simulink model "pfb_fir_16k_4tap_v3_core"  (Simulink 7.8)
settings: Solver=ode45  StartTime=0.0  StopTime=10.0  RelTol=1e-3
libraries: xbsIndex_r4 x287, casper_library_misc x8
(part 1 of 9)
settings Model: Creator=dan  LastModifiedBy=dan
settings DebuggingCC: FcnCallInpInsideContextMsg=Use local settings  StrictBusMsg=Warning

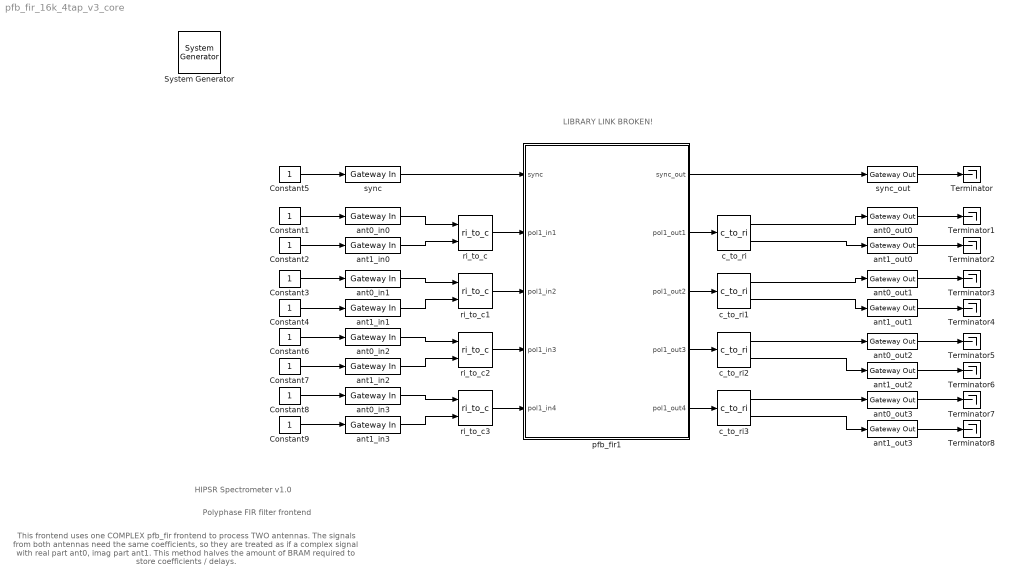
== system pfb_fir_16k_4tap_v3_core ==
  note: Polyphase FIR filter frontend
  note: HIPSR Spectrometer v1.0
  note: This frontend uses one COMPLEX pfb_fir frontend to process TWO antennas.
      | The signals from both antennas need the same coefficients, so they are
      | treated as if a complex signal with real part ant0, imag part ant1.
      | This method halves the amount of BRAM required to store coefficients / delays.
  note: LIBRARY LINK BROKEN!
  " System Generator" : xbsIndex_r4/ System Generator  Tag=genX  xilinxfamily=virtex5  part=xc5vsx95t  speed=-1  package=ff1136  synthesis_tool=XST  clock_wrapper=Clock Enables  directory=/designs/dan/parkes/bb/xb_pfb_fir_16k_4tap_core  proj_type=Project Navigator  Synth_file=XST Defaults  Impl_file=ISE Defaults  testbench=off  simulink_period=1  sysclk_period=10  dcm_input_clock_period=10  incr_netlist=off  trim_vbits=Everywhere in SubSystem  dbl_ovrd=According to Block Masks  core_generation=According to Block Masks  run_coregen=off  deprecated_control=off  eval_field=0  block_type=sysgen
      settings: block_version=11.4
  Constant{1..9} (9 alike) : Constant
  Terminator{,1..8} (9 alike) : Terminator
  ant0_in{0..3} (4 alike) : xbsIndex_r4/Gateway In  gui_display_data_type=Fixed-point  arith_type="Signed  (2's comp)"  n_bits=8  bin_pt=7  preci_type=Single  exp_width=8  frac_width=24  quantization="Round  (unbiased: +/- Inf)"  overflow=Saturate  period=1  dbl_ovrd=off  timing_constraint=None  locs_specified=off  LOCs={}  inherit_from_input=off  UseAsADC=off  ADCChannel='1'  hdl_port=on  block_type=gatewayin
      settings: infoedit="Gateway in block.  Converts inputs of type Simulink integer, double and fixed point to  Xilinx fixed point type.<br><br>Hardware notes:  In hardware these blocks become top level input ports."  block_version=11.4
  ant0_out{0..3} (4 alike) : xbsIndex_r4/Gateway Out  inherit_from_input=off  hdl_port=on  timing_constraint=None  locs_specified=off  LOCs={}  UseAsDAC=off  DACChannel='1'  block_type=gatewayout
      settings: infoedit="Gateway out block.  Converts Xilinx fixed point inputs into ouputs of type Simulink integer, double, or fixed point.<br><br>Hardware notes:  In hardware these blocks become top level output ports or are discarded, depending on how they are configured."  block_version=11.4
  ant1_in{0..3} (4 alike) : xbsIndex_r4/Gateway In  gui_display_data_type=Fixed-point  arith_type="Signed  (2's comp)"  n_bits=8  bin_pt=7  preci_type=Single  exp_width=8  frac_width=24  quantization="Round  (unbiased: +/- Inf)"  overflow=Saturate  period=1  dbl_ovrd=off  timing_constraint=None  locs_specified=off  LOCs={}  inherit_from_input=off  UseAsADC=off  ADCChannel='1'  hdl_port=on  block_type=gatewayin
      settings: infoedit="Gateway in block.  Converts inputs of type Simulink integer, double and fixed point to  Xilinx fixed point type.<br><br>Hardware notes:  In hardware these blocks become top level input ports."  block_version=11.4
  ant1_out{0..3} (4 alike) : xbsIndex_r4/Gateway Out  inherit_from_input=off  hdl_port=on  timing_constraint=None  locs_specified=off  LOCs={}  UseAsDAC=off  DACChannel='1'  block_type=gatewayout
      settings: infoedit="Gateway out block.  Converts Xilinx fixed point inputs into ouputs of type Simulink integer, double, or fixed point.<br><br>Hardware notes:  In hardware these blocks become top level output ports or are discarded, depending on how they are configured."  block_version=11.4
  c_to_ri{,1..3} (4 alike) : casper_library_misc/c_to_ri  n_bits=18  bin_pt=17
  pfb_fir1 : Subsystem  AncestorBlock=xblocks_library_pfbs/pfb_fir  mask(pfb_fir){PFBSize=14, TotalTaps=4, WindowType=hamming, n_inputs=2, MakeBiplex=off, BitWidthIn=8, BitWidthOut=18, CoeffBitWidth=18, CoeffDistMem=off, add_latency=2, mult_latency=3, bram_latency=3, quantization=Round  (unbiased: +/- Inf), fwidth=1, specify_mult=off, mult_spec=[2                                      2]}
      mask prompts: PFBSize "Size of PFB: (2^? pnts)"; TotalTaps "Total Number of Taps:"; WindowType "Windowing Function:"; n_inputs "Number of Simultaneous Inputs: (2^?)"; MakeBiplex "Make Biplex"; BitWidthIn "Input Bitwidth:"; BitWidthOut "Output Bitwidth:"; CoeffBitWidth "Coefficient Bitwidth:"; CoeffDistMem "Use Distributed Memory for Coeffs"; add_latency "Add Latency"; mult_latency "Mult Latency"; bram_latency "BRAM Latency"; quantization "Quantization Behavior"; fwidth "Bin Width Scaling (normal=1)"; specify_mult "Specify multiplier use (behavioral if not specified)"; mult_spec "Multiplier specification (0=core, 1=embedded, 2=behavioural) (left=1st tap)"
      mask init:
      | config.source = str2func('pfb_fir_init_xblock');
      | config.toplevel = gcb;
      | config.depend = get_dependlist('pfb_fir');
      | set_param(gcb,'LinkStatus','inactive');
      | xBlock(config,{config.toplevel, ...
      |     'PFBSize', PFBSize, ...
      |     'TotalTaps', TotalTaps, ...
      |     'WindowType', WindowType, ...
      |     'n_inputs', n_inputs, ...
      |     'MakeBiplex', MakeBiplex, ...
      |     'BitWidthIn', BitWidthIn, ...
      |     'BitWidthOut', BitWidthOut, ...
      |     'CoeffBitWidth', CoeffBitWidth, ...
      |     'CoeffDistMem', CoeffDistMem, ...
      |     'add_latency', add_latency, ...
      |     'mult_latency', mult_latency, ...
      |     'bram_latency', bram_latency, ...
      |     'quantization', quantization, ...
      |     'fwidth', fwidth,...
      |     'specify_mult', specify_mult,...
      |     'mult_spec', mult_spec});
      settings: AttributesFormatString=taps=4, add_latency=2
      mask Help: eval('xlWeb(''http://casper.berkeley.edu/wiki/Pfb_fir'')')
      mask StyleString: edit,edit,popup(bartlett|barthannwin|blackman|blackmanharris|bohamwin|chebwin|flattopwin|gausswin|hamming|hann|kaiser|nuttallwin|parzenwin|rectwin|tukeywin|triang|userwindow),edit,checkbox,edit,edit,edit,checkbox,edit,edit,edit,popup(Truncate|Round  (unbiased: +/- Inf)|Round  (unbiased: Even Values)),edit,checkbox,edit
      mask CallbackString:
      | |%num_taps = eval(get_param(gcb, 'TotalTaps'));
      | %old_vec = eval(get_param(gcb, 'mult_spec'));
      | 
      | %vec = 2.*ones(1,num_taps);
      | %old_size = length(old_vec);
      | 
      | %if(old_size <= num_taps),
      | %   new_size = old_size;
      | %else,
      | %    new_size = num_taps;
      | %end
      | 
      | %for n = 1:new_size, vec(n) = old_vec(n); end
      | %set_param(gcb, 'mult_spec', mat2str(vec));||||||||||||%num_taps = eval(get_param(gcb, 'TotalTaps'));
      | %old_vec = eval(get_param(gcb, 'mult_spec'));
      | 
      | %vec = 2.*ones(1,num_taps);
      | %old_size = length(old_vec);
      | 
      | %if(old_size <= num_taps),
      | %    new_size = old_size;
      | %else,
      | %    new_size = num_taps;
      | %end
      | 
      | %for n = 1:new_size, vec(n) = old_vec(n); end
      | %set_param(gcb, 'mult_spec', mat2str(vec));|%specify_mult = get_param(gcb,'specify_mult');
      | %if( strcmp(specify_mult,'off')),
      | %    set_param(gcb, 'MaskEnables', {'on','on','on','on','on','on','on','on','on','on','on','on','on','on','on','off'});
      | %else
      | %    set_param(gcb, 'MaskEnables', {'on','on','on','on','on','on','on','on','on','on','on','on','on','on','on','on'});
      | %end
      | 
      | |%specify_mult = get_param(gcb,'specify_mult');
      | %if( strcmp(specify_mult,'off')),
      | %    set_param(gcb, 'MaskEnables', {'on','on','on','on','on','on','on','on','on','on','on','on','on','on','on','off'});
      | %else
      | %    set_param(gcb, 'MaskEnables', {'on','on','on','on','on','on','on','on','on','on','on','on','on','on','on','on'});
      | %end
  ri_to_c{,1..3} (4 alike) : casper_library_misc/ri_to_c
  sync : xbsIndex_r4/Gateway In  gui_display_data_type=Fixed-point  arith_type=Boolean  n_bits=16  bin_pt=14  preci_type=Single  exp_width=8  frac_width=24  quantization="Round  (unbiased: +/- Inf)"  overflow=Saturate  period=1  dbl_ovrd=off  timing_constraint=None  locs_specified=off  LOCs={}  inherit_from_input=off  UseAsADC=off  ADCChannel='1'  hdl_port=on  block_type=gatewayin
      settings: infoedit="Gateway in block.  Converts inputs of type Simulink integer, double and fixed point to  Xilinx fixed point type.<br><br>Hardware notes:  In hardware these blocks become top level input ports."  block_version=11.4
  sync_out : xbsIndex_r4/Gateway Out  inherit_from_input=off  hdl_port=on  timing_constraint=None  locs_specified=off  LOCs={}  UseAsDAC=off  DACChannel='1'  block_type=gatewayout
      settings: infoedit="Gateway out block.  Converts Xilinx fixed point inputs into ouputs of type Simulink integer, double, or fixed point.<br><br>Hardware notes:  In hardware these blocks become top level output ports or are discarded, depending on how they are configured."  block_version=11.4
  wires:
  sync/1 -> pfb_fir1/1(sync)
  ri_to_c/1 -> pfb_fir1/2(pol1_in1)
  ri_to_c1/1 -> pfb_fir1/3(pol1_in2)
  ant0_in0/1 -> ri_to_c/1
  Constant5/1 -> sync/1
  Constant1/1 -> ant0_in0/1
  ant1_in0/1 -> ri_to_c/2
  ant0_in1/1 -> ri_to_c1/1
  ant1_in1/1 -> ri_to_c1/2
  Constant4/1 -> ant1_in1/1
  Constant3/1 -> ant0_in1/1
  Constant2/1 -> ant1_in0/1
  pfb_fir1/2(pol1_out1) -> c_to_ri/1
  pfb_fir1/3(pol1_out2) -> c_to_ri1/1
  sync_out/1 -> Terminator/1
  ant1_out0/1 -> Terminator2/1
  ant0_out0/1 -> Terminator1/1
  ant0_in2/1 -> ri_to_c2/1
  ant1_in2/1 -> ri_to_c2/2
  Constant7/1 -> ant1_in2/1
  Constant6/1 -> ant0_in2/1
  ant0_in3/1 -> ri_to_c3/1
  ant1_in3/1 -> ri_to_c3/2
  Constant9/1 -> ant1_in3/1
  Constant8/1 -> ant0_in3/1
  ri_to_c2/1 -> pfb_fir1/4(pol1_in3)
  ri_to_c3/1 -> pfb_fir1/5(pol1_in4)
  pfb_fir1/1(sync_out) -> sync_out/1
  ant1_out1/1 -> Terminator4/1
  ant0_out1/1 -> Terminator3/1
  ant1_out2/1 -> Terminator6/1
  ant0_out2/1 -> Terminator5/1
  ant1_out3/1 -> Terminator8/1
  ant0_out3/1 -> Terminator7/1
  c_to_ri/1 -> ant0_out0/1
  c_to_ri/2 -> ant1_out0/1
  c_to_ri1/1 -> ant0_out1/1
  c_to_ri1/2 -> ant1_out1/1
  c_to_ri2/1 -> ant0_out2/1
  c_to_ri2/2 -> ant1_out2/1
  c_to_ri3/1 -> ant0_out3/1
  c_to_ri3/2 -> ant1_out3/1
  pfb_fir1/4(pol1_out3) -> c_to_ri2/1
  pfb_fir1/5(pol1_out4) -> c_to_ri3/1

== system pfb_fir_16k_4tap_v3_core/pfb_fir1 ==
  sync : Inport
  pol1_in1 : Inport  Port=2
  pol1_in2 : Inport  Port=3
  pol1_in3 : Inport  Port=4
  pol1_in4 : Inport  Port=5
  pfb_row_11 : Subsystem
  pfb_row_12 : Subsystem
  pfb_row_13 : Subsystem
  pfb_row_14 : Subsystem
  sync_out : Outport
  pol1_out1 : Outport  Port=2
  pol1_out2 : Outport  Port=3
  pol1_out3 : Outport  Port=4
  pol1_out4 : Outport  Port=5
  wires:
  sync/1 -> pfb_row_14/2(sync), pfb_row_13/2(sync), pfb_row_12/2(sync), pfb_row_11/2(sync)
  pfb_row_14/2(out) -> pol1_out4/1
  pol1_in4/1 -> pfb_row_14/1(din)
  pfb_row_13/2(out) -> pol1_out3/1
  pol1_in3/1 -> pfb_row_13/1(din)
  pfb_row_12/2(out) -> pol1_out2/1
  pol1_in2/1 -> pfb_row_12/1(din)
  pfb_row_11/2(out) -> pol1_out1/1
  pfb_row_11/1(sync_out) -> sync_out/1
  pol1_in1/1 -> pfb_row_11/1(din)

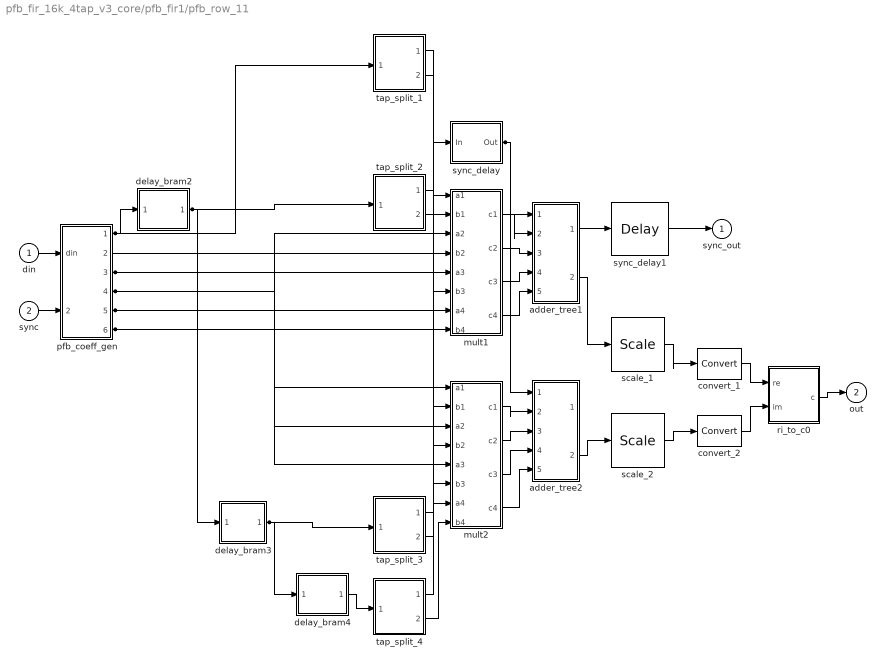
== system pfb_fir_16k_4tap_v3_core/pfb_fir1/pfb_row_11 ==
  din : Inport
  sync : Inport  Port=2
  adder_tree1 : Subsystem
  adder_tree2 : Subsystem
  convert_1 : xbsIndex_r4/Convert  gui_display_data_type=Fixed-point  arith_type="Signed  (2's comp)"  n_bits=18  bin_pt=17  float_type=Single  exp_bits=8  fraction_bits=24  quantization="Round  (unbiased: +/- Inf)"  overflow=Saturate  en=off  latency=3  dbl_ovrd=off  pipeline=on  block_type=convert
  convert_2 : xbsIndex_r4/Convert  gui_display_data_type=Fixed-point  arith_type="Signed  (2's comp)"  n_bits=18  bin_pt=17  float_type=Single  exp_bits=8  fraction_bits=24  quantization="Round  (unbiased: +/- Inf)"  overflow=Saturate  en=off  latency=3  dbl_ovrd=off  pipeline=on  block_type=convert
  delay_bram2 : Subsystem
  delay_bram3 : Subsystem
  delay_bram4 : Subsystem
  mult1 : Subsystem
  mult2 : Subsystem
  pfb_coeff_gen : Subsystem
      settings: AttributesFormatString=PFBSize=14, n_inputs=2, taps=4
  ri_to_c0 : Subsystem
  scale_1 : xbsIndex_r4/Scale  scale_factor=-3  dbl_ovrd=off  block_type=scale
  scale_2 : xbsIndex_r4/Scale  scale_factor=-3  dbl_ovrd=off  block_type=scale
  sync_delay : Subsystem
  sync_delay1 : xbsIndex_r4/Delay  rst=off  infoeditControl=Selection of Reset will increase slice count due to use of real FFs and instead of SRLs  en=off  latency=3  dbl_ovrd=off  reg_retiming=off  block_type=delay
  tap_split_1 : Subsystem
      settings: AttributesFormatString=Fix_8_7
  tap_split_2 : Subsystem
      settings: AttributesFormatString=Fix_8_7
  tap_split_3 : Subsystem
      settings: AttributesFormatString=Fix_8_7
  tap_split_4 : Subsystem
      settings: AttributesFormatString=Fix_8_7
  sync_out : Outport
  out : Outport  Port=2
  wires:
  pfb_coeff_gen/1(dout) -> tap_split_1/1(inport), delay_bram2/1(din_1_1)
  delay_bram2/1(dout_1_1) -> tap_split_2/1(inport), delay_bram3/1(din_1_1)
  delay_bram3/1(dout_1_1) -> tap_split_3/1(inport), delay_bram4/1(din_1_1)
  pfb_coeff_gen/3(coeffs1) -> mult2/1(a1), mult1/1(a1)
  pfb_coeff_gen/4(coeffs2) -> mult2/3(a2), mult1/3(a2)
  pfb_coeff_gen/5(coeffs3) -> mult2/5(a3), mult1/5(a3)
  pfb_coeff_gen/6(coeffs4) -> mult2/7(a4), mult1/7(a4)
  sync_delay/1(Out) -> adder_tree2/1(sync), adder_tree1/1(sync)
  ri_to_c0/1(c) -> out/1
  convert_2/1 -> ri_to_c0/2(im)
  convert_1/1 -> ri_to_c0/1(re)
  scale_2/1 -> convert_2/1
  adder_tree2/2(dout) -> scale_2/1
  mult2/4(c4) -> adder_tree2/5(din_4)
  mult2/3(c3) -> adder_tree2/4(din_3)
  mult2/2(c2) -> adder_tree2/3(din_2)
  mult2/1(c1) -> adder_tree2/2(din_1)
  tap_split_4/2(outport2) -> mult2/8(b4)
  tap_split_3/2(outport2) -> mult2/6(b3)
  tap_split_2/2(outport2) -> mult2/4(b2)
  tap_split_1/2(outport2) -> mult2/2(b1)
  sync_delay1/1 -> sync_out/1
  adder_tree1/1(sync_out) -> sync_delay1/1
  scale_1/1 -> convert_1/1
  adder_tree1/2(dout) -> scale_1/1
  mult1/4(c4) -> adder_tree1/5(din_4)
  mult1/3(c3) -> adder_tree1/4(din_3)
  mult1/2(c2) -> adder_tree1/3(din_2)
  mult1/1(c1) -> adder_tree1/2(din_1)
  tap_split_4/1(outport1) -> mult1/8(b4)
  tap_split_3/1(outport1) -> mult1/6(b3)
  tap_split_2/1(outport1) -> mult1/4(b2)
  tap_split_1/1(outport1) -> mult1/2(b1)
  delay_bram4/1(dout_1_1) -> tap_split_4/1(inport)
  pfb_coeff_gen/2(sync_out) -> sync_delay/1(In)
  sync/1 -> pfb_coeff_gen/2(sync)
  din/1 -> pfb_coeff_gen/1(din)

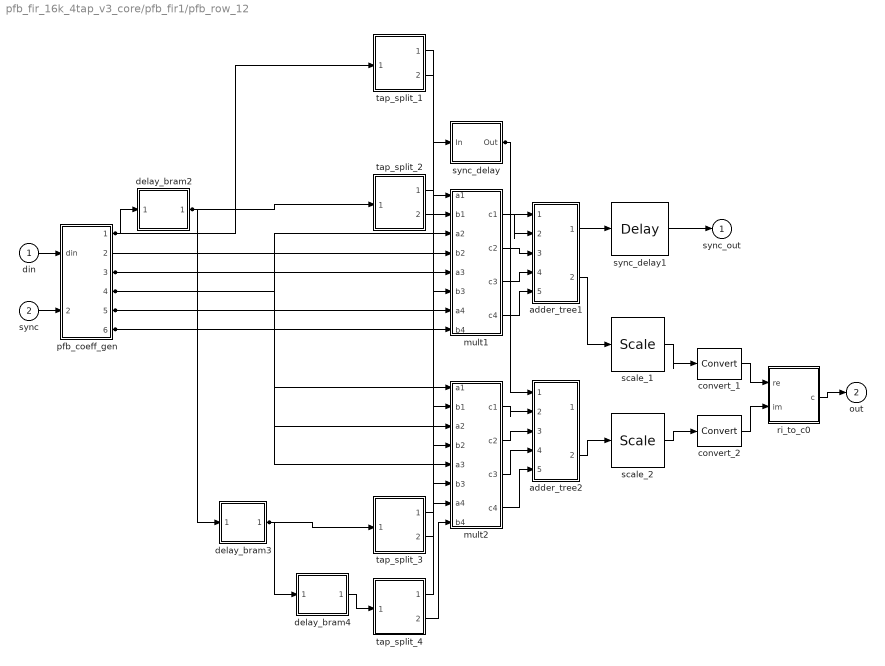
== system pfb_fir_16k_4tap_v3_core/pfb_fir1/pfb_row_12 ==
  din : Inport
  sync : Inport  Port=2
  adder_tree1 : Subsystem
  adder_tree2 : Subsystem
  convert_1 : xbsIndex_r4/Convert  gui_display_data_type=Fixed-point  arith_type="Signed  (2's comp)"  n_bits=18  bin_pt=17  float_type=Single  exp_bits=8  fraction_bits=24  quantization="Round  (unbiased: +/- Inf)"  overflow=Saturate  en=off  latency=3  dbl_ovrd=off  pipeline=on  block_type=convert
  convert_2 : xbsIndex_r4/Convert  gui_display_data_type=Fixed-point  arith_type="Signed  (2's comp)"  n_bits=18  bin_pt=17  float_type=Single  exp_bits=8  fraction_bits=24  quantization="Round  (unbiased: +/- Inf)"  overflow=Saturate  en=off  latency=3  dbl_ovrd=off  pipeline=on  block_type=convert
  delay_bram2 : Subsystem
  delay_bram3 : Subsystem
  delay_bram4 : Subsystem
  mult1 : Subsystem
  mult2 : Subsystem
  pfb_coeff_gen : Subsystem
      settings: AttributesFormatString=PFBSize=14, n_inputs=2, taps=4
  ri_to_c0 : Subsystem
  scale_1 : xbsIndex_r4/Scale  scale_factor=-3  dbl_ovrd=off  block_type=scale
  scale_2 : xbsIndex_r4/Scale  scale_factor=-3  dbl_ovrd=off  block_type=scale
  sync_delay : Subsystem
  sync_delay1 : xbsIndex_r4/Delay  rst=off  infoeditControl=Selection of Reset will increase slice count due to use of real FFs and instead of SRLs  en=off  latency=3  dbl_ovrd=off  reg_retiming=off  block_type=delay
  tap_split_1 : Subsystem
      settings: AttributesFormatString=Fix_8_7
  tap_split_2 : Subsystem
      settings: AttributesFormatString=Fix_8_7
  tap_split_3 : Subsystem
      settings: AttributesFormatString=Fix_8_7
  tap_split_4 : Subsystem
      settings: AttributesFormatString=Fix_8_7
  sync_out : Outport
  out : Outport  Port=2
  wires:
  pfb_coeff_gen/1(dout) -> tap_split_1/1(inport), delay_bram2/1(din_1_1)
  delay_bram2/1(dout_1_1) -> tap_split_2/1(inport), delay_bram3/1(din_1_1)
  delay_bram3/1(dout_1_1) -> tap_split_3/1(inport), delay_bram4/1(din_1_1)
  pfb_coeff_gen/3(coeffs1) -> mult2/1(a1), mult1/1(a1)
  pfb_coeff_gen/4(coeffs2) -> mult2/3(a2), mult1/3(a2)
  pfb_coeff_gen/5(coeffs3) -> mult2/5(a3), mult1/5(a3)
  pfb_coeff_gen/6(coeffs4) -> mult2/7(a4), mult1/7(a4)
  sync_delay/1(Out) -> adder_tree2/1(sync), adder_tree1/1(sync)
  ri_to_c0/1(c) -> out/1
  convert_2/1 -> ri_to_c0/2(im)
  convert_1/1 -> ri_to_c0/1(re)
  scale_2/1 -> convert_2/1
  adder_tree2/2(dout) -> scale_2/1
  mult2/4(c4) -> adder_tree2/5(din_4)
  mult2/3(c3) -> adder_tree2/4(din_3)
  mult2/2(c2) -> adder_tree2/3(din_2)
  mult2/1(c1) -> adder_tree2/2(din_1)
  tap_split_4/2(outport2) -> mult2/8(b4)
  tap_split_3/2(outport2) -> mult2/6(b3)
  tap_split_2/2(outport2) -> mult2/4(b2)
  tap_split_1/2(outport2) -> mult2/2(b1)
  sync_delay1/1 -> sync_out/1
  adder_tree1/1(sync_out) -> sync_delay1/1
  scale_1/1 -> convert_1/1
  adder_tree1/2(dout) -> scale_1/1
  mult1/4(c4) -> adder_tree1/5(din_4)
  mult1/3(c3) -> adder_tree1/4(din_3)
  mult1/2(c2) -> adder_tree1/3(din_2)
  mult1/1(c1) -> adder_tree1/2(din_1)
  tap_split_4/1(outport1) -> mult1/8(b4)
  tap_split_3/1(outport1) -> mult1/6(b3)
  tap_split_2/1(outport1) -> mult1/4(b2)
  tap_split_1/1(outport1) -> mult1/2(b1)
  delay_bram4/1(dout_1_1) -> tap_split_4/1(inport)
  pfb_coeff_gen/2(sync_out) -> sync_delay/1(In)
  sync/1 -> pfb_coeff_gen/2(sync)
  din/1 -> pfb_coeff_gen/1(din)

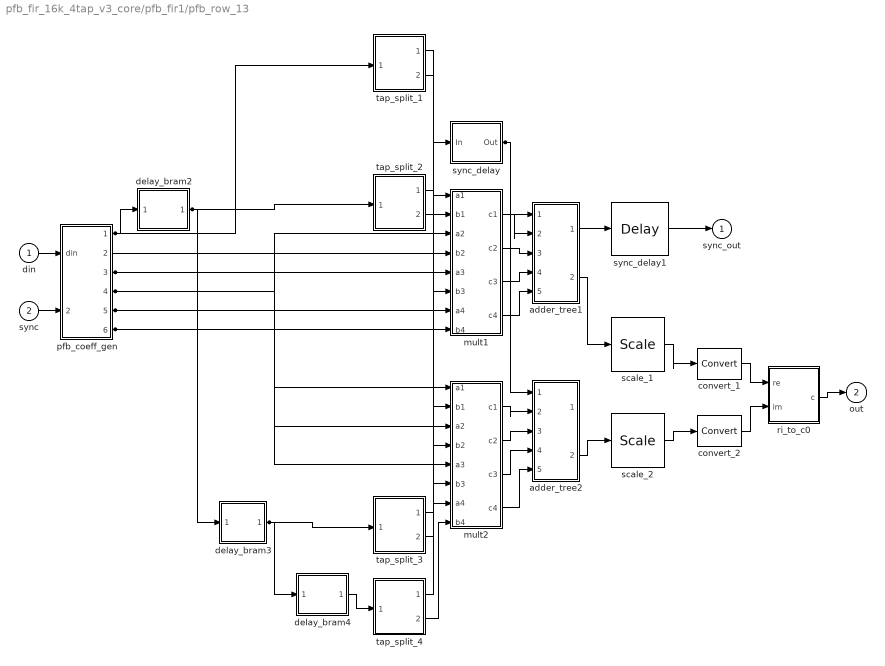
== system pfb_fir_16k_4tap_v3_core/pfb_fir1/pfb_row_13 ==
  din : Inport
  sync : Inport  Port=2
  adder_tree1 : Subsystem
  adder_tree2 : Subsystem
  convert_1 : xbsIndex_r4/Convert  gui_display_data_type=Fixed-point  arith_type="Signed  (2's comp)"  n_bits=18  bin_pt=17  float_type=Single  exp_bits=8  fraction_bits=24  quantization="Round  (unbiased: +/- Inf)"  overflow=Saturate  en=off  latency=3  dbl_ovrd=off  pipeline=on  block_type=convert
  convert_2 : xbsIndex_r4/Convert  gui_display_data_type=Fixed-point  arith_type="Signed  (2's comp)"  n_bits=18  bin_pt=17  float_type=Single  exp_bits=8  fraction_bits=24  quantization="Round  (unbiased: +/- Inf)"  overflow=Saturate  en=off  latency=3  dbl_ovrd=off  pipeline=on  block_type=convert
  delay_bram2 : Subsystem
  delay_bram3 : Subsystem
  delay_bram4 : Subsystem
  mult1 : Subsystem
  mult2 : Subsystem
  pfb_coeff_gen : Subsystem
      settings: AttributesFormatString=PFBSize=14, n_inputs=2, taps=4
  ri_to_c0 : Subsystem
  scale_1 : xbsIndex_r4/Scale  scale_factor=-3  dbl_ovrd=off  block_type=scale
  scale_2 : xbsIndex_r4/Scale  scale_factor=-3  dbl_ovrd=off  block_type=scale
  sync_delay : Subsystem
  sync_delay1 : xbsIndex_r4/Delay  rst=off  infoeditControl=Selection of Reset will increase slice count due to use of real FFs and instead of SRLs  en=off  latency=3  dbl_ovrd=off  reg_retiming=off  block_type=delay
  tap_split_1 : Subsystem
      settings: AttributesFormatString=Fix_8_7
  tap_split_2 : Subsystem
      settings: AttributesFormatString=Fix_8_7
  tap_split_3 : Subsystem
      settings: AttributesFormatString=Fix_8_7
  tap_split_4 : Subsystem
      settings: AttributesFormatString=Fix_8_7
  sync_out : Outport
  out : Outport  Port=2
  wires:
  pfb_coeff_gen/1(dout) -> tap_split_1/1(inport), delay_bram2/1(din_1_1)
  delay_bram2/1(dout_1_1) -> tap_split_2/1(inport), delay_bram3/1(din_1_1)
  delay_bram3/1(dout_1_1) -> tap_split_3/1(inport), delay_bram4/1(din_1_1)
  pfb_coeff_gen/3(coeffs1) -> mult2/1(a1), mult1/1(a1)
  pfb_coeff_gen/4(coeffs2) -> mult2/3(a2), mult1/3(a2)
  pfb_coeff_gen/5(coeffs3) -> mult2/5(a3), mult1/5(a3)
  pfb_coeff_gen/6(coeffs4) -> mult2/7(a4), mult1/7(a4)
  sync_delay/1(Out) -> adder_tree2/1(sync), adder_tree1/1(sync)
  ri_to_c0/1(c) -> out/1
  convert_2/1 -> ri_to_c0/2(im)
  convert_1/1 -> ri_to_c0/1(re)
  scale_2/1 -> convert_2/1
  adder_tree2/2(dout) -> scale_2/1
  mult2/4(c4) -> adder_tree2/5(din_4)
  mult2/3(c3) -> adder_tree2/4(din_3)
  mult2/2(c2) -> adder_tree2/3(din_2)
  mult2/1(c1) -> adder_tree2/2(din_1)
  tap_split_4/2(outport2) -> mult2/8(b4)
  tap_split_3/2(outport2) -> mult2/6(b3)
  tap_split_2/2(outport2) -> mult2/4(b2)
  tap_split_1/2(outport2) -> mult2/2(b1)
  sync_delay1/1 -> sync_out/1
  adder_tree1/1(sync_out) -> sync_delay1/1
  scale_1/1 -> convert_1/1
  adder_tree1/2(dout) -> scale_1/1
  mult1/4(c4) -> adder_tree1/5(din_4)
  mult1/3(c3) -> adder_tree1/4(din_3)
  mult1/2(c2) -> adder_tree1/3(din_2)
  mult1/1(c1) -> adder_tree1/2(din_1)
  tap_split_4/1(outport1) -> mult1/8(b4)
  tap_split_3/1(outport1) -> mult1/6(b3)
  tap_split_2/1(outport1) -> mult1/4(b2)
  tap_split_1/1(outport1) -> mult1/2(b1)
  delay_bram4/1(dout_1_1) -> tap_split_4/1(inport)
  pfb_coeff_gen/2(sync_out) -> sync_delay/1(In)
  sync/1 -> pfb_coeff_gen/2(sync)
  din/1 -> pfb_coeff_gen/1(din)

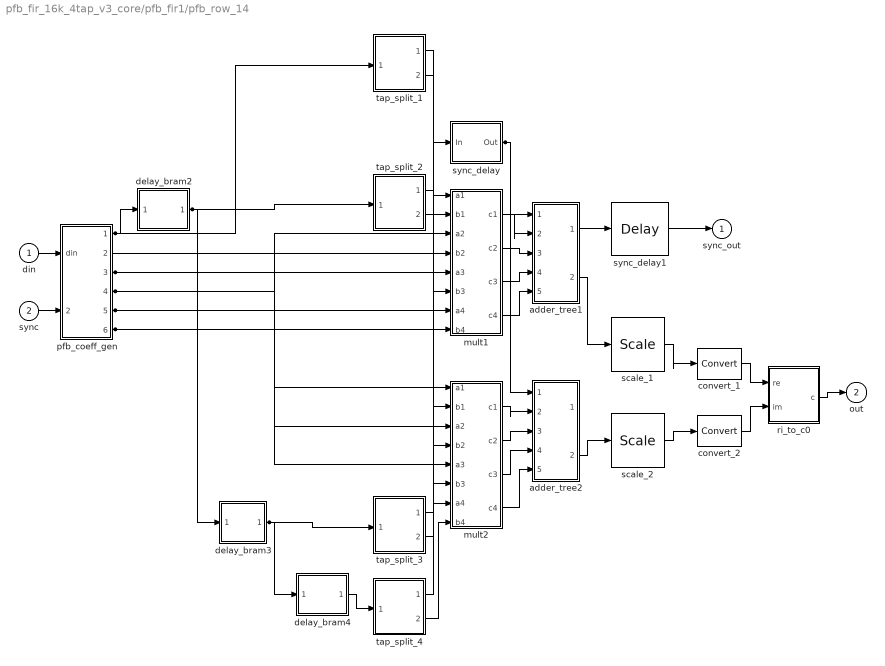
== system pfb_fir_16k_4tap_v3_core/pfb_fir1/pfb_row_14 ==
  din : Inport
  sync : Inport  Port=2
  adder_tree1 : Subsystem
  adder_tree2 : Subsystem
  convert_1 : xbsIndex_r4/Convert  gui_display_data_type=Fixed-point  arith_type="Signed  (2's comp)"  n_bits=18  bin_pt=17  float_type=Single  exp_bits=8  fraction_bits=24  quantization="Round  (unbiased: +/- Inf)"  overflow=Saturate  en=off  latency=3  dbl_ovrd=off  pipeline=on  block_type=convert
  convert_2 : xbsIndex_r4/Convert  gui_display_data_type=Fixed-point  arith_type="Signed  (2's comp)"  n_bits=18  bin_pt=17  float_type=Single  exp_bits=8  fraction_bits=24  quantization="Round  (unbiased: +/- Inf)"  overflow=Saturate  en=off  latency=3  dbl_ovrd=off  pipeline=on  block_type=convert
  delay_bram2 : Subsystem
  delay_bram3 : Subsystem
  delay_bram4 : Subsystem
  mult1 : Subsystem
  mult2 : Subsystem
  pfb_coeff_gen : Subsystem
      settings: AttributesFormatString=PFBSize=14, n_inputs=2, taps=4
  ri_to_c0 : Subsystem
  scale_1 : xbsIndex_r4/Scale  scale_factor=-3  dbl_ovrd=off  block_type=scale
  scale_2 : xbsIndex_r4/Scale  scale_factor=-3  dbl_ovrd=off  block_type=scale
  sync_delay : Subsystem
  sync_delay1 : xbsIndex_r4/Delay  rst=off  infoeditControl=Selection of Reset will increase slice count due to use of real FFs and instead of SRLs  en=off  latency=3  dbl_ovrd=off  reg_retiming=off  block_type=delay
  tap_split_1 : Subsystem
      settings: AttributesFormatString=Fix_8_7
  tap_split_2 : Subsystem
      settings: AttributesFormatString=Fix_8_7
  tap_split_3 : Subsystem
      settings: AttributesFormatString=Fix_8_7
  tap_split_4 : Subsystem
      settings: AttributesFormatString=Fix_8_7
  sync_out : Outport
  out : Outport  Port=2
  wires:
  pfb_coeff_gen/1(dout) -> tap_split_1/1(inport), delay_bram2/1(din_1_1)
  delay_bram2/1(dout_1_1) -> tap_split_2/1(inport), delay_bram3/1(din_1_1)
  delay_bram3/1(dout_1_1) -> tap_split_3/1(inport), delay_bram4/1(din_1_1)
  pfb_coeff_gen/3(coeffs1) -> mult2/1(a1), mult1/1(a1)
  pfb_coeff_gen/4(coeffs2) -> mult2/3(a2), mult1/3(a2)
  pfb_coeff_gen/5(coeffs3) -> mult2/5(a3), mult1/5(a3)
  pfb_coeff_gen/6(coeffs4) -> mult2/7(a4), mult1/7(a4)
  sync_delay/1(Out) -> adder_tree2/1(sync), adder_tree1/1(sync)
  ri_to_c0/1(c) -> out/1
  convert_2/1 -> ri_to_c0/2(im)
  convert_1/1 -> ri_to_c0/1(re)
  scale_2/1 -> convert_2/1
  adder_tree2/2(dout) -> scale_2/1
  mult2/4(c4) -> adder_tree2/5(din_4)
  mult2/3(c3) -> adder_tree2/4(din_3)
  mult2/2(c2) -> adder_tree2/3(din_2)
  mult2/1(c1) -> adder_tree2/2(din_1)
  tap_split_4/2(outport2) -> mult2/8(b4)
  tap_split_3/2(outport2) -> mult2/6(b3)
  tap_split_2/2(outport2) -> mult2/4(b2)
  tap_split_1/2(outport2) -> mult2/2(b1)
  sync_delay1/1 -> sync_out/1
  adder_tree1/1(sync_out) -> sync_delay1/1
  scale_1/1 -> convert_1/1
  adder_tree1/2(dout) -> scale_1/1
  mult1/4(c4) -> adder_tree1/5(din_4)
  mult1/3(c3) -> adder_tree1/4(din_3)
  mult1/2(c2) -> adder_tree1/3(din_2)
  mult1/1(c1) -> adder_tree1/2(din_1)
  tap_split_4/1(outport1) -> mult1/8(b4)
  tap_split_3/1(outport1) -> mult1/6(b3)
  tap_split_2/1(outport1) -> mult1/4(b2)
  tap_split_1/1(outport1) -> mult1/2(b1)
  delay_bram4/1(dout_1_1) -> tap_split_4/1(inport)
  pfb_coeff_gen/2(sync_out) -> sync_delay/1(In)
  sync/1 -> pfb_coeff_gen/2(sync)
  din/1 -> pfb_coeff_gen/1(din)

== system pfb_fir_16k_4tap_v3_core/pfb_fir1/pfb_row_11/adder_tree1 ==
  sync : Inport
  din_1 : Inport  Port=2
  din_2 : Inport  Port=3
  din_3 : Inport  Port=4
  din_4 : Inport  Port=5
  adder_0 : xbsIndex_r4/AddSub  mode=Addition  use_carryin=off  use_carryout=off  en=off  latency=2  precision=Full  arith_type=Unsigned  n_bits=18  bin_pt=17  quantization="Round  (unbiased: +/- Inf)"  overflow=Wrap  dbl_ovrd=off  use_behavioral_HDL=on  hw_selection=Fabric  pipelined=off  block_type=addsub
  adder_1 : xbsIndex_r4/AddSub  mode=Addition  use_carryin=off  use_carryout=off  en=off  latency=2  precision=Full  arith_type=Unsigned  n_bits=18  bin_pt=17  quantization="Round  (unbiased: +/- Inf)"  overflow=Wrap  dbl_ovrd=off  use_behavioral_HDL=on  hw_selection=Fabric  pipelined=off  block_type=addsub
  adder_2 : xbsIndex_r4/AddSub  mode=Addition  use_carryin=off  use_carryout=off  en=off  latency=2  precision=Full  arith_type=Unsigned  n_bits=18  bin_pt=17  quantization="Round  (unbiased: +/- Inf)"  overflow=Wrap  dbl_ovrd=off  use_behavioral_HDL=on  hw_selection=Fabric  pipelined=off  block_type=addsub
  sync_delay : xbsIndex_r4/Delay  rst=off  infoeditControl=Selection of Reset will increase slice count due to use of real FFs and instead of SRLs  en=off  latency=4  dbl_ovrd=off  reg_retiming=off  block_type=delay
  sync_out : Outport
  dout : Outport  Port=2
  wires:
  adder_2/1 -> dout/1
  adder_0/1 -> adder_2/2
  adder_1/1 -> adder_2/1
  din_3/1 -> adder_1/2
  din_4/1 -> adder_1/1
  din_1/1 -> adder_0/2
  din_2/1 -> adder_0/1
  sync_delay/1 -> sync_out/1
  sync/1 -> sync_delay/1

== system pfb_fir_16k_4tap_v3_core/pfb_fir1/pfb_row_11/adder_tree2 ==
  sync : Inport
  din_1 : Inport  Port=2
  din_2 : Inport  Port=3
  din_3 : Inport  Port=4
  din_4 : Inport  Port=5
  adder_0 : xbsIndex_r4/AddSub  mode=Addition  use_carryin=off  use_carryout=off  en=off  latency=2  precision=Full  arith_type=Unsigned  n_bits=18  bin_pt=17  quantization="Round  (unbiased: +/- Inf)"  overflow=Wrap  dbl_ovrd=off  use_behavioral_HDL=on  hw_selection=Fabric  pipelined=off  block_type=addsub
  adder_1 : xbsIndex_r4/AddSub  mode=Addition  use_carryin=off  use_carryout=off  en=off  latency=2  precision=Full  arith_type=Unsigned  n_bits=18  bin_pt=17  quantization="Round  (unbiased: +/- Inf)"  overflow=Wrap  dbl_ovrd=off  use_behavioral_HDL=on  hw_selection=Fabric  pipelined=off  block_type=addsub
  adder_2 : xbsIndex_r4/AddSub  mode=Addition  use_carryin=off  use_carryout=off  en=off  latency=2  precision=Full  arith_type=Unsigned  n_bits=18  bin_pt=17  quantization="Round  (unbiased: +/- Inf)"  overflow=Wrap  dbl_ovrd=off  use_behavioral_HDL=on  hw_selection=Fabric  pipelined=off  block_type=addsub
  sync_delay : xbsIndex_r4/Delay  rst=off  infoeditControl=Selection of Reset will increase slice count due to use of real FFs and instead of SRLs  en=off  latency=4  dbl_ovrd=off  reg_retiming=off  block_type=delay
  sync_out : Outport
  dout : Outport  Port=2
  wires:
  adder_2/1 -> dout/1
  adder_0/1 -> adder_2/2
  adder_1/1 -> adder_2/1
  din_3/1 -> adder_1/2
  din_4/1 -> adder_1/1
  din_1/1 -> adder_0/2
  din_2/1 -> adder_0/1
  sync_delay/1 -> sync_out/1
  sync/1 -> sync_delay/1

== system pfb_fir_16k_4tap_v3_core/pfb_fir1/pfb_row_11/delay_bram2 ==
  din_1_1 : Inport
  Constant1 : xbsIndex_r4/Constant  const=0  gui_display_data_type=Fixed-point  arith_type=Unsigned  n_bits=2  bin_pt=0  preci_type=Single  exp_width=8  frac_width=24  explicit_period=on  period=1  equ=P=C  opselect=C  inp2=PCIN>>17  opr=+  inp1=P  carry=CIN  dbl_ovrd=off  block_type=constant
  Constant2 : xbsIndex_r4/Constant  const=1  gui_display_data_type=Fixed-point  arith_type=Boolean  n_bits=1  bin_pt=0  preci_type=Single  exp_width=8  frac_width=24  explicit_period=on  period=1  equ=P=C  opselect=C  inp2=PCIN>>17  opr=+  inp1=P  carry=CIN  dbl_ovrd=off  block_type=constant
  bram1 : xbsIndex_r4/Single Port RAM  depth=4  initVector=0  distributed_mem=Block RAM  write_mode=Read Before Write  rst=off  init_reg=0  en=off  latency=4  dbl_ovrd=off  optimize=Area  use_rpm=off  block_type=spram
  dout_1_1 : Outport
  wires:
  bram1/1 -> dout_1_1/1
  Constant2/1 -> bram1/3
  din_1_1/1 -> bram1/2
  Constant1/1 -> bram1/1

== system pfb_fir_16k_4tap_v3_core/pfb_fir1/pfb_row_11/delay_bram3 ==
  din_1_1 : Inport
  Constant1 : xbsIndex_r4/Constant  const=0  gui_display_data_type=Fixed-point  arith_type=Unsigned  n_bits=2  bin_pt=0  preci_type=Single  exp_width=8  frac_width=24  explicit_period=on  period=1  equ=P=C  opselect=C  inp2=PCIN>>17  opr=+  inp1=P  carry=CIN  dbl_ovrd=off  block_type=constant
  Constant2 : xbsIndex_r4/Constant  const=1  gui_display_data_type=Fixed-point  arith_type=Boolean  n_bits=1  bin_pt=0  preci_type=Single  exp_width=8  frac_width=24  explicit_period=on  period=1  equ=P=C  opselect=C  inp2=PCIN>>17  opr=+  inp1=P  carry=CIN  dbl_ovrd=off  block_type=constant
  bram1 : xbsIndex_r4/Single Port RAM  depth=4  initVector=0  distributed_mem=Block RAM  write_mode=Read Before Write  rst=off  init_reg=0  en=off  latency=4  dbl_ovrd=off  optimize=Area  use_rpm=off  block_type=spram
  dout_1_1 : Outport
  wires:
  bram1/1 -> dout_1_1/1
  Constant2/1 -> bram1/3
  din_1_1/1 -> bram1/2
  Constant1/1 -> bram1/1

== system pfb_fir_16k_4tap_v3_core/pfb_fir1/pfb_row_11/delay_bram4 ==
  din_1_1 : Inport
  Constant1 : xbsIndex_r4/Constant  const=0  gui_display_data_type=Fixed-point  arith_type=Unsigned  n_bits=2  bin_pt=0  preci_type=Single  exp_width=8  frac_width=24  explicit_period=on  period=1  equ=P=C  opselect=C  inp2=PCIN>>17  opr=+  inp1=P  carry=CIN  dbl_ovrd=off  block_type=constant
  Constant2 : xbsIndex_r4/Constant  const=1  gui_display_data_type=Fixed-point  arith_type=Boolean  n_bits=1  bin_pt=0  preci_type=Single  exp_width=8  frac_width=24  explicit_period=on  period=1  equ=P=C  opselect=C  inp2=PCIN>>17  opr=+  inp1=P  carry=CIN  dbl_ovrd=off  block_type=constant
  bram1 : xbsIndex_r4/Single Port RAM  depth=4  initVector=0  distributed_mem=Block RAM  write_mode=Read Before Write  rst=off  init_reg=0  en=off  latency=4  dbl_ovrd=off  optimize=Area  use_rpm=off  block_type=spram
  dout_1_1 : Outport
  wires:
  bram1/1 -> dout_1_1/1
  Constant2/1 -> bram1/3
  din_1_1/1 -> bram1/2
  Constant1/1 -> bram1/1

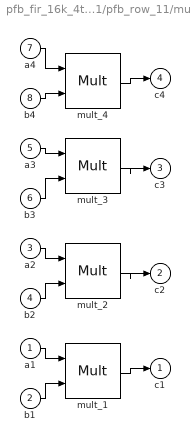
== system pfb_fir_16k_4tap_v3_core/pfb_fir1/pfb_row_11/mult1 ==
  a1 : Inport
  b1 : Inport  Port=2
  a2 : Inport  Port=3
  b2 : Inport  Port=4
  a3 : Inport  Port=5
  b3 : Inport  Port=6
  a4 : Inport  Port=7
  b4 : Inport  Port=8
  mult_{1..4} (4 alike) : xbsIndex_r4/Mult  precision=Full  arith_type="Signed  (2's comp)"  n_bits=16  bin_pt=14  quantization=Truncate  overflow=Wrap  en=off  latency=3  dbl_ovrd=off  use_behavioral_HDL=off  opt=Speed  use_embedded=on  optimum_pipeline=off  pipeline=on  use_rpm=on  placement_style=Triangular  block_type=mult
  c1 : Outport
  c2 : Outport  Port=2
  c3 : Outport  Port=3
  c4 : Outport  Port=4
  wires:
  mult_4/1 -> c4/1
  b4/1 -> mult_4/2
  a4/1 -> mult_4/1
  mult_3/1 -> c3/1
  b3/1 -> mult_3/2
  a3/1 -> mult_3/1
  mult_2/1 -> c2/1
  b2/1 -> mult_2/2
  a2/1 -> mult_2/1
  mult_1/1 -> c1/1
  b1/1 -> mult_1/2
  a1/1 -> mult_1/1

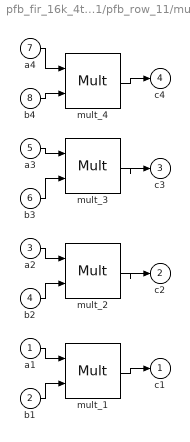
== system pfb_fir_16k_4tap_v3_core/pfb_fir1/pfb_row_11/mult2 ==
  a1 : Inport
  b1 : Inport  Port=2
  a2 : Inport  Port=3
  b2 : Inport  Port=4
  a3 : Inport  Port=5
  b3 : Inport  Port=6
  a4 : Inport  Port=7
  b4 : Inport  Port=8
  mult_{1..4} (4 alike) : xbsIndex_r4/Mult  precision=Full  arith_type="Signed  (2's comp)"  n_bits=16  bin_pt=14  quantization=Truncate  overflow=Wrap  en=off  latency=3  dbl_ovrd=off  use_behavioral_HDL=off  opt=Speed  use_embedded=on  optimum_pipeline=off  pipeline=on  use_rpm=on  placement_style=Triangular  block_type=mult
  c1 : Outport
  c2 : Outport  Port=2
  c3 : Outport  Port=3
  c4 : Outport  Port=4
  wires:
  mult_4/1 -> c4/1
  b4/1 -> mult_4/2
  a4/1 -> mult_4/1
  mult_3/1 -> c3/1
  b3/1 -> mult_3/2
  a3/1 -> mult_3/1
  mult_2/1 -> c2/1
  b2/1 -> mult_2/2
  a2/1 -> mult_2/1
  mult_1/1 -> c1/1
  b1/1 -> mult_1/2
  a1/1 -> mult_1/1
